simulink model "Torque_controller"  (R2023b)
settings: Solver=VariableStepAuto  StartTime=0.0  StopTime=50  RelTol=1e-3
values from neighbouring files (symbols this model uses):
  b = (1/windowSize)*ones(1,windowSize)    [attempt.m]    (also in model_approximation.m; torque.m = 0.016; tuning.m)
  Im = 0.059    [torque.m]
  k = 0.85    [torque.m]
  Ki = 5049.4    [torque.m]
  Kp = 5049.4*0.01    (= 50.494)    [torque.m]
  L = [l1;l2;l3]    [observer.m]    (also in torque.m = 0.0082)
  R = 0.01    [attempt.m]    (also in controller_tuning.m = 0.08; progetto.m = 0.001; torque.m = 3.2; tuning.m = 0.001)
settings Model: Creator=giova  LastModifiedBy=david

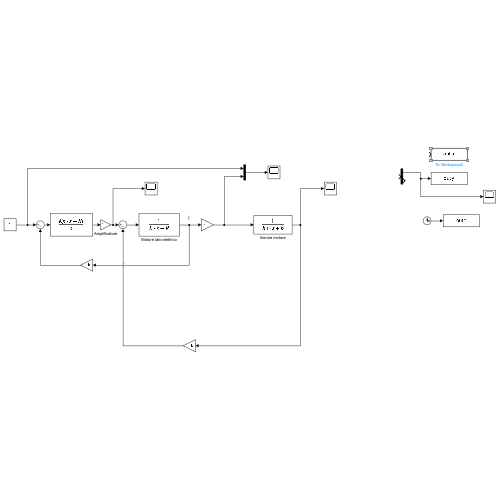
[thumbnail: Simulink's stored preview of the top-level diagram]
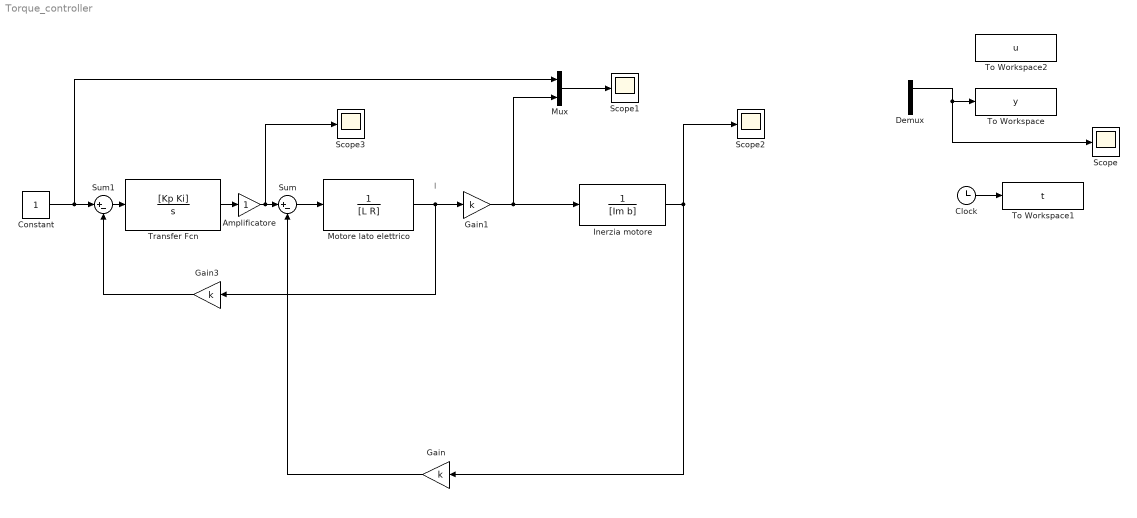
== system Torque_controller ==
  note: I
  Amplificatore : Gain
  Clock : Clock
  Constant : Constant
  Demux : Demux  Outputs=2
  Gain : Gain  Gain=k
  Gain1 : Gain  Gain=k
  Gain3 : Gain  Gain=k
  Inerzia motore : TransferFcn  Denominator=[Im b]
  Motore lato elettrico : TransferFcn  Denominator=[L R]
  Mux : Mux  Inputs=2
  Scope{,1..3} (4 alike) : Scope
  Sum : Sum  Inputs=|+-
  Sum1 : Sum  Inputs=|+-
  To Workspace : ToWorkspace  VariableName=y  SampleTime=-1
  To Workspace1 : ToWorkspace  VariableName=t  SampleTime=-1
  To Workspace2 : ToWorkspace  VariableName=u  SampleTime=-1
  Transfer Fcn : TransferFcn  Numerator=[Kp Ki]  Denominator=[1 0]
  wires:
  Clock/1 -> To Workspace1/1
  Demux/1 -> Scope/1, To Workspace/1
  Gain1/1 -> Mux/2, Inerzia motore/1
  Motore lato elettrico/1 -> Gain1/1, Gain3/1
  Sum/1 -> Motore lato elettrico/1
  Inerzia motore/1 -> Gain/1, Scope2/1
  Gain/1 -> Sum/2
  Constant/1 -> Mux/1, Sum1/1
  Mux/1 -> Scope1/1
  Sum1/1 -> Transfer Fcn/1
  Transfer Fcn/1 -> Amplificatore/1
  Amplificatore/1 -> Scope3/1, Sum/1
  Gain3/1 -> Sum1/2
